simulink model "p1"  (R2023a)
settings: Solver=VariableStepAuto  StartTime=0.0  StopTime=10.0  RelTol=1e-3
model workspace (MAT data in the model file):
  X = 1
settings Model: Creator=Amirali  LastModifiedBy=Amirali

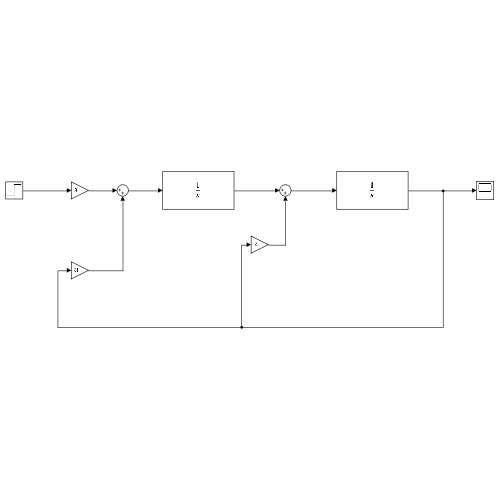
[thumbnail: Simulink's stored preview of the top-level diagram]
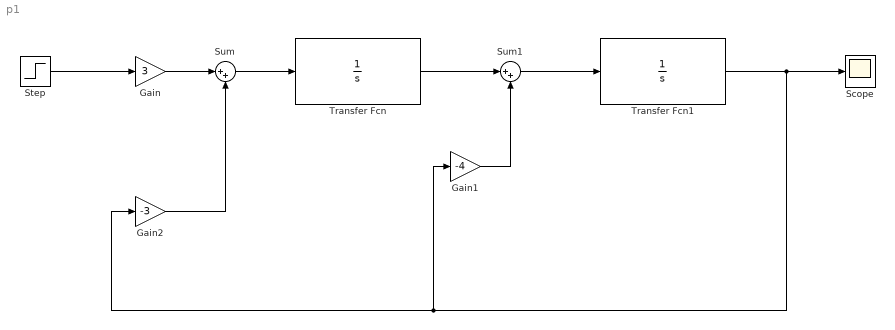
== system p1 ==
  Gain : Gain  Gain=3
  Gain1 : Gain  Gain=-4
  Gain2 : Gain  Gain=-3
  Scope : Scope
  Step : Step  SampleTime=0
  Sum : Sum  Inputs=|++
  Sum1 : Sum  Inputs=|++
  Transfer Fcn : TransferFcn  Denominator=[1 0]
  Transfer Fcn1 : TransferFcn  Denominator=[1 0]
  wires:
  Gain/1 -> Sum/1
  Sum/1 -> Transfer Fcn/1
  Transfer Fcn/1 -> Sum1/1
  Sum1/1 -> Transfer Fcn1/1
  Gain2/1 -> Sum/2
  Transfer Fcn1/1 -> Gain1/1, Gain2/1, Scope/1
  Gain1/1 -> Sum1/2
  Step/1 -> Gain/1
